simulink model "ADRC_model"  (Simulink 7.6)
settings: Solver=ode45  StartTime=0.0  StopTime=50  RelTol=1e-3
libraries: ADRC x3
settings Model: Creator=Administrator  LastModifiedBy=Administrator
settings DebuggingCC: AlgebraicLoopMsg=none  ArtificialAlgebraicLoopMsg=none  SolverPrmCheckMsg=none  UnknownTsInhSupMsg=none

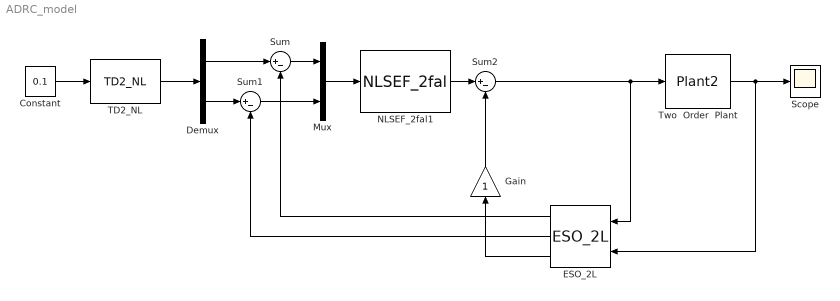
== system ADRC_model ==
  Constant : Constant  Value=0.1
  Demux : Demux  Outputs=2
  ESO_2L : ADRC/ESO/ESO_2L/ESO_2L  SystemSampleTime=-1  bet=[100 65 82]  b=1
  Gain : Gain
  Mux : Mux  Inputs=2
  NLSEF_2fal1 : ADRC/SEF/NLSEF/NLSEF_2fal  Beta1=8  Beta2=5  A1=0.25  A2=0.5  Delta=0.1
  Scope : Scope
      settings: YMin=-1.2e+019  YMax=0
  Sum : Sum  Inputs=|+-
  Sum1 : Sum  Inputs=|+-
  Sum2 : Sum  Inputs=|+-
  TD2_NL : ADRC/TD/TD2_NL/TD2_NL  r=1  h=0.1  h0=0.1
  Two  Order  Plant : S-Function  FunctionName=Plant2  EnableBusSupport=off
  wires:
  Constant/1 -> TD2_NL/1
  TD2_NL/1 -> Demux/1
  Demux/1 -> Sum/1
  Demux/2 -> Sum1/1
  ESO_2L/1 -> Sum/2
  ESO_2L/2 -> Sum1/2
  Sum/1 -> Mux/1
  Sum1/1 -> Mux/2
  Mux/1 -> NLSEF_2fal1/1
  Two  Order  Plant/1 -> Scope/1, ESO_2L/2
  ESO_2L/3 -> Gain/1
  NLSEF_2fal1/1 -> Sum2/1
  Gain/1 -> Sum2/2
  Sum2/1 -> Two  Order  Plant/1, ESO_2L/1
